simulink model "1"  (R2019a)
settings: Solver=VariableStepAuto  StartTime=0.0  StopTime=10.0  RelTol=1e-3
values from neighbouring files (symbols this model uses):
  C = 1    [value.m]
  J = 1    [value.m]
  K1 = 1    [value.m]
  K2 = 1    [value.m]
  L = 1    [value.m]
  R = 1    [value.m]
settings Model: Creator=TakumiShiota  LastModifiedBy=TakumiShiota

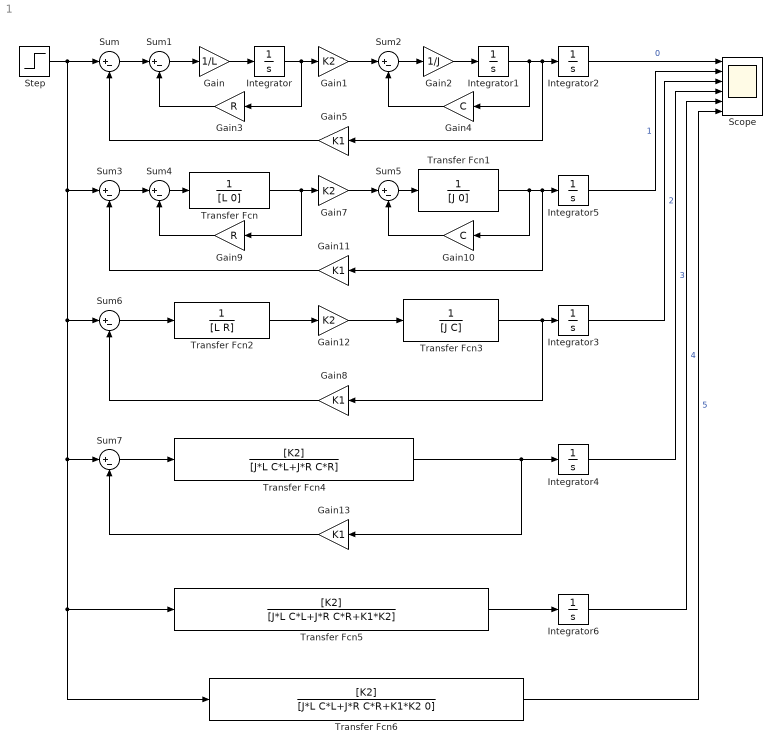
== system 1 ==
  Gain : Gain  Gain=1/L
  Gain1 : Gain  Gain=K2
  Gain10 : Gain  Gain=C
  Gain{5,8,11,13} (4 alike) : Gain  Gain=K1
  Gain12 : Gain  Gain=K2
  Gain2 : Gain  Gain=1/J
  Gain3 : Gain  Gain=R
  Gain4 : Gain  Gain=C
  Gain7 : Gain  Gain=K2
  Gain9 : Gain  Gain=R
  Integrator{,1..6} (7 alike) : Integrator
  Scope : Scope  NumInputPorts=6
  Step : Step  SampleTime=0
  Sum{,1..7} (8 alike) : Sum  Inputs=|+-
  Transfer Fcn : TransferFcn  Denominator=[L 0]
  Transfer Fcn1 : TransferFcn  Denominator=[J 0]
  Transfer Fcn2 : TransferFcn  Denominator=[L R]
  Transfer Fcn3 : TransferFcn  Denominator=[J C]
  Transfer Fcn4 : TransferFcn  Numerator=[K2]  Denominator=[J*L C*L+J*R C*R]
  Transfer Fcn5 : TransferFcn  Numerator=[K2]  Denominator=[J*L C*L+J*R C*R+K1*K2]
  Transfer Fcn6 : TransferFcn  Numerator=[K2]  Denominator=[J*L C*L+J*R C*R+K1*K2 0]
  wires:
  Sum1/1 -> Gain/1
  Gain/1 -> Integrator/1
  Integrator/1 -> Gain3/1, Gain1/1
  Gain1/1 -> Sum2/1
  Sum2/1 -> Gain2/1
  Gain2/1 -> Integrator1/1
  Integrator1/1 -> Gain4/1, Gain5/1, Integrator2/1
  Sum/1 -> Sum1/1
  Gain4/1 -> Sum2/2
  Gain3/1 -> Sum1/2
  Gain5/1 -> Sum/2
  Integrator2/1 -> Scope/1  "0"
  Gain11/1 -> Sum3/2
  Sum3/1 -> Sum4/1
  Transfer Fcn1/1 -> Gain10/1, Gain11/1, Integrator5/1
  Gain10/1 -> Sum5/2
  Transfer Fcn/1 -> Gain9/1, Gain7/1
  Gain9/1 -> Sum4/2
  Gain7/1 -> Sum5/1
  Integrator5/1 -> Scope/2  "1"
  Sum4/1 -> Transfer Fcn/1
  Sum5/1 -> Transfer Fcn1/1
  Transfer Fcn3/1 -> Gain8/1, Integrator3/1
  Sum6/1 -> Transfer Fcn2/1
  Transfer Fcn2/1 -> Gain12/1
  Gain8/1 -> Sum6/2
  Gain12/1 -> Transfer Fcn3/1
  Integrator3/1 -> Scope/3  "2"
  Gain13/1 -> Sum7/2
  Sum7/1 -> Transfer Fcn4/1
  Transfer Fcn4/1 -> Integrator4/1, Gain13/1
  Integrator4/1 -> Scope/4  "3"
  Step/1 -> Transfer Fcn6/1, Transfer Fcn5/1, Sum7/1, Sum6/1, Sum3/1, Sum/1
  Transfer Fcn5/1 -> Integrator6/1
  Integrator6/1 -> Scope/5  "4"
  Transfer Fcn6/1 -> Scope/6  "5"
